simulink library "QuadModelLib"  (R2023a)
settings: Solver=VariableStepAuto  StartTime=0.0  StopTime=10.0  RelTol=1e-3
values from neighbouring files (symbols this model uses):
  ModelParam_envAltitude = -50    [Init.m]
  ModelParam_noisePowerIMU = 0    [Init.m]
  ModelParam_timeSampBaro = 0.01    [Init.m]
  MotorFault1 = MotorFaultTemp    [Init.m]
undefined symbols (not defined in the file or in its folder): BatteryFault, Earth, F, FaultParamAPI, Light, LoadFault, MIL, ModelParam_noiseLowPassFilterCoeAccel, ModelParam_noiseLowPassFilterCoeGyro, Moderate, PropFault, SensorFault, WGS84, WindFault
libraries: aerolibwind2 x4, aerolibtransform2 x1, simulink x1, aerolibasang x1, aerolibatmos2 x1, aerolibnav x1, aerolibgravity2 x1
(part 1 of 2)
settings Model: Creator=dream  LastModifiedBy=RFLYSIM
settings SolverCC: AlgebraicLoopSolver=TrustRegion
settings DataIOCC: ReturnWorkspaceOutputs=off
settings DebuggingCC: UnconnectedInputMsg=warning  UnconnectedOutputMsg=warning  UnconnectedLineMsg=warning  ArithmeticOperatorsInVariantConditions=warning
settings ModelReferenceCC: EnableRefExpFcnMdlSchedulingChecks=on
settings SFSimCC: SimUseLocalCustomCode=off  CustomCodeUndefinedFunction=UseInterfaceOnly
settings RTWCC: RTWUseLocalCustomCode=off  DLArmComputeVersion=19.05

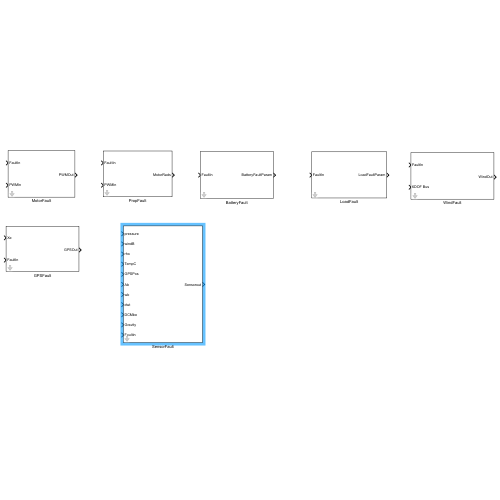
[thumbnail: Simulink's stored preview of the top-level diagram]
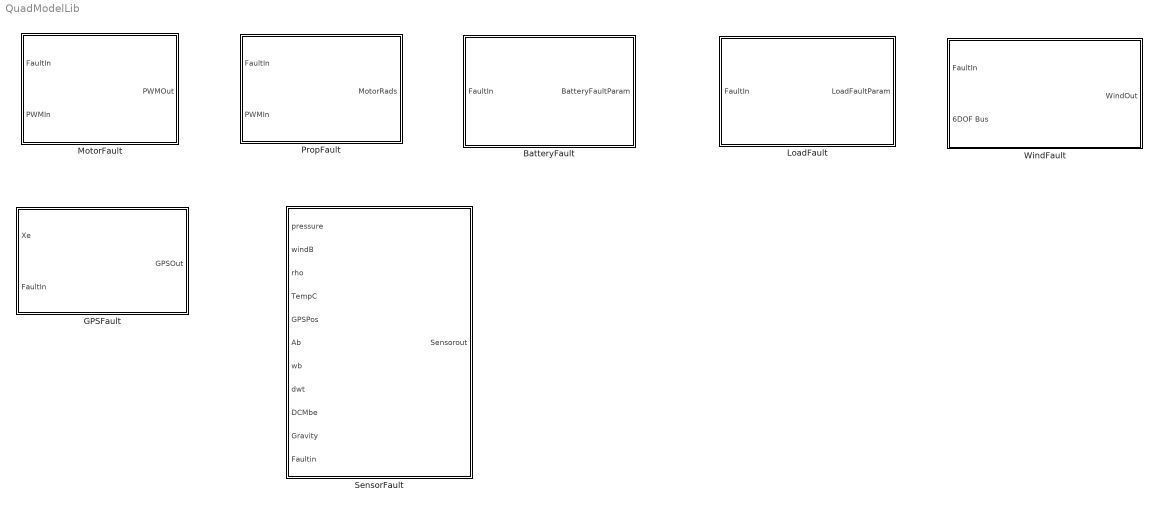
== system QuadModelLib ==
  BatteryFault : Subsystem  mask{FaultParamStruct=BatteryFault}
      mask prompts: FaultParamStruct "Fault Param Struct"
  GPSFault : Subsystem  mask{FaultParamStruct=SensorFault}
      mask prompts: FaultParamStruct "Fault Param Struct"
  LoadFault : Subsystem  mask{FaultParamStruct=LoadFault}
      mask prompts: FaultParamStruct "Fault Param Struct"
  MotorFault : Subsystem  mask{FaultParamStruct=MotorFault1, ComParamVect=FaultParamAPI}
      mask prompts: FaultParamStruct "Fault Param Struct"; ComParamVect "Common Param Vect"
  PropFault : Subsystem  mask{FaultParamStruct=PropFault, ComParamVect=FaultParamAPI}
      mask prompts: FaultParamStruct "Fault Param Struct"; ComParamVect "Common Struct Vect"
  SensorFault : Subsystem  mask{FaultParamStruct=SensorFault, ComParamVect=FaultParamAPI}
      mask prompts: FaultParamStruct "Fault Param Struct"; ComParamVect "Common Param Vect"
  WindFault : Subsystem  mask{FaultParamStruct=WindFault, ComParamVect=FaultParamAPI}
      mask prompts: FaultParamStruct "Fault Param Struct"; ComParamVect "Common Param Vect"

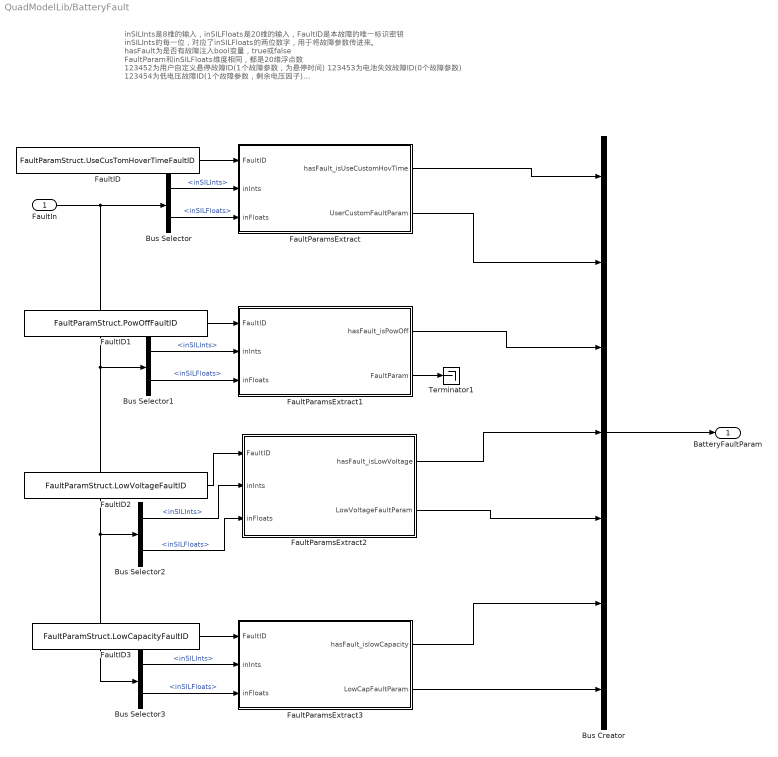
== system QuadModelLib/BatteryFault ==
  note: inSILInts是8维的输入，inSILFloats是20维的输入，FaultID是本故障的唯一标识密钥
      | inSILInts的每一位，对应了inSILFloats的两位数字，用于将故障参数传进来。
      |
      | hasFault为是否有故障注入bool变量，true或false
      | FaultParam和inSILFloats维度相同，都是20维浮点数
      |
      | 123452为用户自定义悬停故障ID(1个故障参数，为悬停时间)
      | 123453为电池失效故障ID(0个故障参数)
      | 123454为低电压故障ID(1个故障参数，剩余电压因子)
      | 123455为低电量故障ID(1个故障参数，剩余电量因子)
      |
      | 注：如果没有新的故障注入进来，FaultParamsExtract会保持上一时刻的值。
  FaultIn : Inport
  Bus Creator : BusCreator  Inputs=7
  Bus Selector{,1..3} (4 alike) : BusSelector  OutputSignals=inSILInts,inSILFloats
  FaultID : Constant  Value=FaultParamStruct.UseCusTomHoverTimeFaultID  OutDataTypeStr=int32
  FaultID1 : Constant  Value=FaultParamStruct.PowOffFaultID  OutDataTypeStr=int32
  FaultID2 : Constant  Value=FaultParamStruct.LowVoltageFaultID  OutDataTypeStr=int32
  FaultID3 : Constant  Value=FaultParamStruct.LowCapacityFaultID  OutDataTypeStr=int32
  FaultParamsExtract : MATLAB Function  TreatAsAtomicUnit=on
  FaultParamsExtract1 : MATLAB Function  TreatAsAtomicUnit=on
  FaultParamsExtract2 : MATLAB Function  TreatAsAtomicUnit=on
  FaultParamsExtract3 : MATLAB Function  TreatAsAtomicUnit=on
  Terminator1 : Terminator
  BatteryFaultParam : Outport
  wires:
  Bus Selector3/2 -> FaultParamsExtract3/3(inFloats)  "<inSILFloats>"
  Bus Selector3/1 -> FaultParamsExtract3/2(inInts)  "<inSILInts>"
  FaultIn/1 -> Bus Selector/1, Bus Selector3/1, Bus Selector2/1, Bus Selector1/1
  Bus Selector1/1 -> FaultParamsExtract1/2(inInts)  "<inSILInts>"
  Bus Selector2/1 -> FaultParamsExtract2/2(inInts)  "<inSILInts>"
  FaultParamsExtract2/2(LowVoltageFaultParam) -> Bus Creator/5
  Bus Selector/1 -> FaultParamsExtract/2(inInts)  "<inSILInts>"
  FaultID2/1 -> FaultParamsExtract2/1(FaultID)
  FaultParamsExtract3/2(LowCapFaultParam) -> Bus Creator/7
  Bus Selector1/2 -> FaultParamsExtract1/3(inFloats)  "<inSILFloats>"
  FaultParamsExtract/2(UserCustomFaultParam) -> Bus Creator/2
  FaultID1/1 -> FaultParamsExtract1/1(FaultID)
  FaultID3/1 -> FaultParamsExtract3/1(FaultID)
  Bus Selector2/2 -> FaultParamsExtract2/3(inFloats)  "<inSILFloats>"
  FaultParamsExtract1/2(FaultParam) -> Terminator1/1
  Bus Selector/2 -> FaultParamsExtract/3(inFloats)  "<inSILFloats>"
  FaultID/1 -> FaultParamsExtract/1(FaultID)
  FaultParamsExtract1/1(hasFault_isPowOff) -> Bus Creator/3
  FaultParamsExtract/1(hasFault_isUseCustomHovTime) -> Bus Creator/1
  FaultParamsExtract2/1(hasFault_isLowVoltage) -> Bus Creator/4
  FaultParamsExtract3/1(hasFault_islowCapacity) -> Bus Creator/6
  Bus Creator/1 -> BatteryFaultParam/1

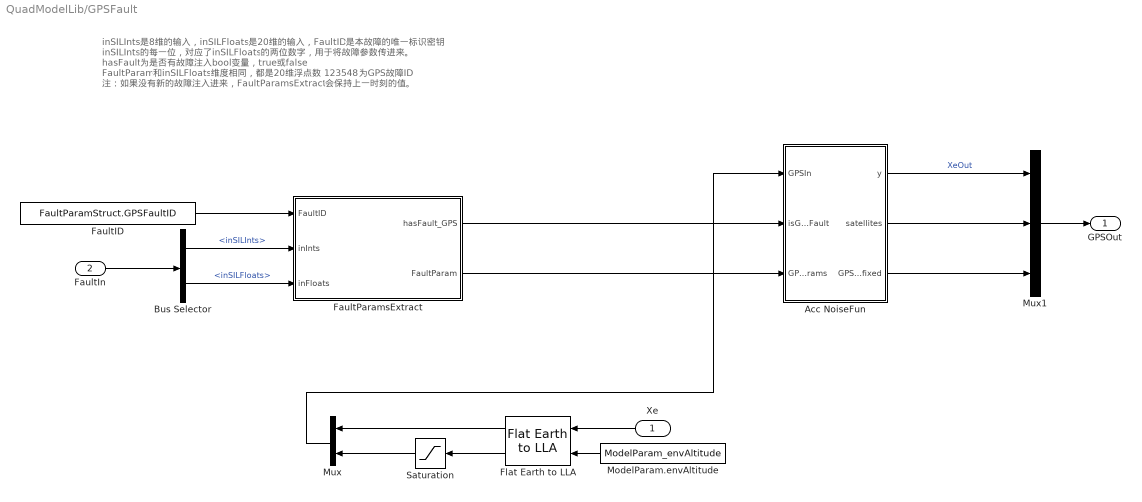
== system QuadModelLib/GPSFault ==
  note: inSILInts是8维的输入，inSILFloats是20维的输入，FaultID是本故障的唯一标识密钥
      | inSILInts的每一位，对应了inSILFloats的两位数字，用于将故障参数传进来。
      |
      | hasFault为是否有故障注入bool变量，true或false
      | FaultParam和inSILFloats维度相同，都是20维浮点数
      |
      | 123548为GPS故障ID
      |
      | 注：如果没有新的故障注入进来，FaultParamsExtract会保持上一时刻的值。
  Xe : Inport
  FaultIn : Inport  Port=2
  Acc NoiseFun : MATLAB Function  TreatAsAtomicUnit=on
  Bus Selector : BusSelector  OutputSignals=inSILInts,inSILFloats
  FaultID : Constant  Value=FaultParamStruct.GPSFaultID  OutDataTypeStr=int32
  FaultParamsExtract : MATLAB Function  TreatAsAtomicUnit=on
  Flat Earth to LLA : aerolibtransform2/Flat Earth to LLA  units=Metric (MKS)  ptype=Earth (WGS84)  F=1/298.257223563  R=6378137  refPosPort=off  LL0=ModelParam_GPSLatLong  psi=0
  ModelParam.envAltitude : Constant  Value=ModelParam_envAltitude
  Mux : Mux  Inputs=2
  Mux1 : Mux  Inputs=3
  Saturation : Saturate  UpperLimit=100000  LowerLimit=0
  GPSOut : Outport
  wires:
  FaultParamsExtract/1(hasFault_GPS) -> Acc NoiseFun/2(isGPSFault)
  Bus Selector/2 -> FaultParamsExtract/3(inFloats)  "<inSILFloats>"
  FaultID/1 -> FaultParamsExtract/1(FaultID)
  FaultIn/1 -> Bus Selector/1
  FaultParamsExtract/2(FaultParam) -> Acc NoiseFun/3(GPSFaultParams)
  Flat Earth to LLA/2 -> Saturation/1
  ModelParam.envAltitude/1 -> Flat Earth to LLA/2
  Flat Earth to LLA/1 -> Mux/1
  Saturation/1 -> Mux/2
  Bus Selector/1 -> FaultParamsExtract/2(inInts)  "<inSILInts>"
  Acc NoiseFun/2(satellites) -> Mux1/2
  Acc NoiseFun/3(GPS3Dfixed) -> Mux1/3
  Mux1/1 -> GPSOut/1
  Xe/1 -> Flat Earth to LLA/1
  Mux/1 -> Acc NoiseFun/1(GPSIn)
  Acc NoiseFun/1(y) -> Mux1/1  "XeOut"

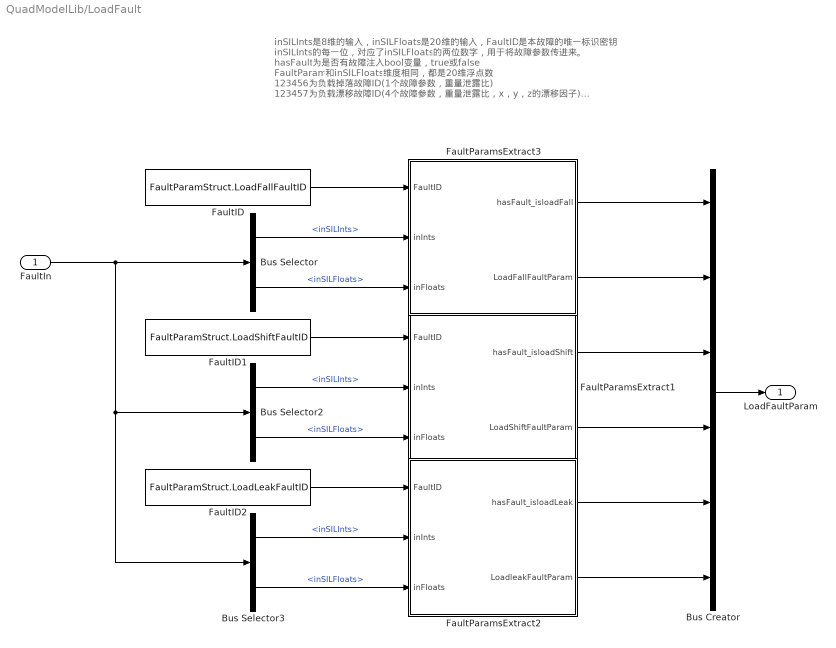
== system QuadModelLib/LoadFault ==
  note: inSILInts是8维的输入，inSILFloats是20维的输入，FaultID是本故障的唯一标识密钥
      | inSILInts的每一位，对应了inSILFloats的两位数字，用于将故障参数传进来。
      |
      | hasFault为是否有故障注入bool变量，true或false
      | FaultParam和inSILFloats维度相同，都是20维浮点数
      |
      | 123456为负载掉落故障ID(1个故障参数，重量泄露比)
      | 123457为负载漂移故障ID(4个故障参数，重量泄露比，x，y，z的漂移因子)
      | 123458为负载泄露故障ID(2个故障参数，1个重量泄露比，1个泄露因子)
      | 注：如果没有新的故障注入进来，FaultParamsExtract会保持上一时刻的值。
  FaultIn : Inport
  Bus Creator : BusCreator  Inputs=6
  Bus Selector : BusSelector  OutputSignals=inSILInts,inSILFloats
  Bus Selector2 : BusSelector  OutputSignals=inSILInts,inSILFloats
  Bus Selector3 : BusSelector  OutputSignals=inSILInts,inSILFloats
  FaultID : Constant  Value=FaultParamStruct.LoadFallFaultID  OutDataTypeStr=int32
  FaultID1 : Constant  Value=FaultParamStruct.LoadShiftFaultID  OutDataTypeStr=int32
  FaultID2 : Constant  Value=FaultParamStruct.LoadLeakFaultID  OutDataTypeStr=int32
  FaultParamsExtract1 : MATLAB Function  TreatAsAtomicUnit=on
  FaultParamsExtract2 : MATLAB Function  TreatAsAtomicUnit=on
  FaultParamsExtract3 : MATLAB Function  TreatAsAtomicUnit=on
  LoadFaultParam : Outport
  wires:
  FaultIn/1 -> Bus Selector3/1, Bus Selector2/1, Bus Selector/1
  Bus Selector3/2 -> FaultParamsExtract2/3(inFloats)  "<inSILFloats>"
  Bus Selector/1 -> FaultParamsExtract3/2(inInts)  "<inSILInts>"
  Bus Selector2/2 -> FaultParamsExtract1/3(inFloats)  "<inSILFloats>"
  Bus Selector3/1 -> FaultParamsExtract2/2(inInts)  "<inSILInts>"
  Bus Selector2/1 -> FaultParamsExtract1/2(inInts)  "<inSILInts>"
  Bus Selector/2 -> FaultParamsExtract3/3(inFloats)  "<inSILFloats>"
  FaultID/1 -> FaultParamsExtract3/1(FaultID)
  FaultID2/1 -> FaultParamsExtract2/1(FaultID)
  FaultID1/1 -> FaultParamsExtract1/1(FaultID)
  FaultParamsExtract3/1(hasFault_isloadFall) -> Bus Creator/1
  FaultParamsExtract3/2(LoadFallFaultParam) -> Bus Creator/2
  FaultParamsExtract1/1(hasFault_isloadShift) -> Bus Creator/3
  FaultParamsExtract1/2(LoadShiftFaultParam) -> Bus Creator/4
  FaultParamsExtract2/1(hasFault_isloadLeak) -> Bus Creator/5
  FaultParamsExtract2/2(LoadleakFaultParam) -> Bus Creator/6
  Bus Creator/1 -> LoadFaultParam/1

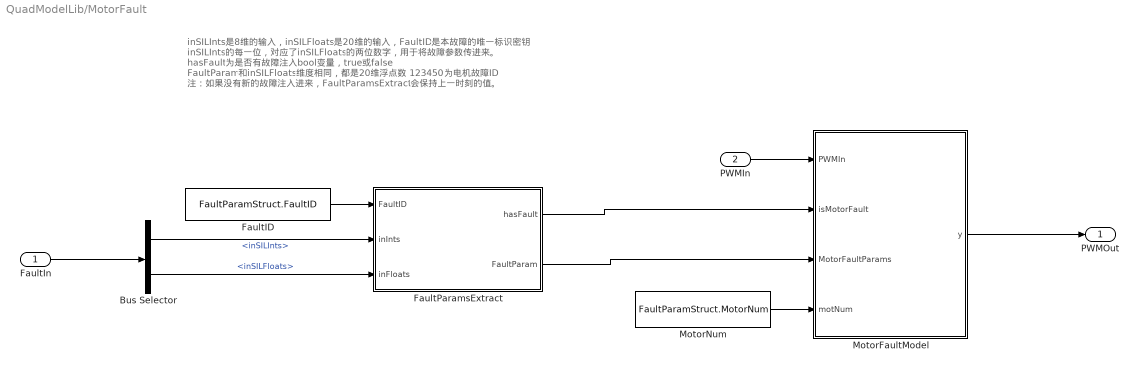
== system QuadModelLib/MotorFault ==
  note: inSILInts是8维的输入，inSILFloats是20维的输入，FaultID是本故障的唯一标识密钥
      | inSILInts的每一位，对应了inSILFloats的两位数字，用于将故障参数传进来。
      |
      | hasFault为是否有故障注入bool变量，true或false
      | FaultParam和inSILFloats维度相同，都是20维浮点数
      |
      | 123450为电机故障ID
      |
      | 注：如果没有新的故障注入进来，FaultParamsExtract会保持上一时刻的值。
  FaultIn : Inport
  PWMIn : Inport  Port=2
  Bus Selector : BusSelector  OutputSignals=inSILInts,inSILFloats
  FaultID : Constant  Value=FaultParamStruct.FaultID  OutDataTypeStr=int32
  FaultParamsExtract : MATLAB Function  TreatAsAtomicUnit=on
  MotorFaultModel : MATLAB Function  TreatAsAtomicUnit=on
  MotorNum : Constant  Value=FaultParamStruct.MotorNum  OutDataTypeStr=int32
  PWMOut : Outport
  wires:
  FaultIn/1 -> Bus Selector/1
  FaultID/1 -> FaultParamsExtract/1(FaultID)
  MotorFaultModel/1(y) -> PWMOut/1
  Bus Selector/2 -> FaultParamsExtract/3(inFloats)  "<inSILFloats>"
  MotorNum/1 -> MotorFaultModel/4(motNum)
  Bus Selector/1 -> FaultParamsExtract/2(inInts)  "<inSILInts>"
  PWMIn/1 -> MotorFaultModel/1(PWMIn)
  FaultParamsExtract/1(hasFault) -> MotorFaultModel/2(isMotorFault)
  FaultParamsExtract/2(FaultParam) -> MotorFaultModel/3(MotorFaultParams)

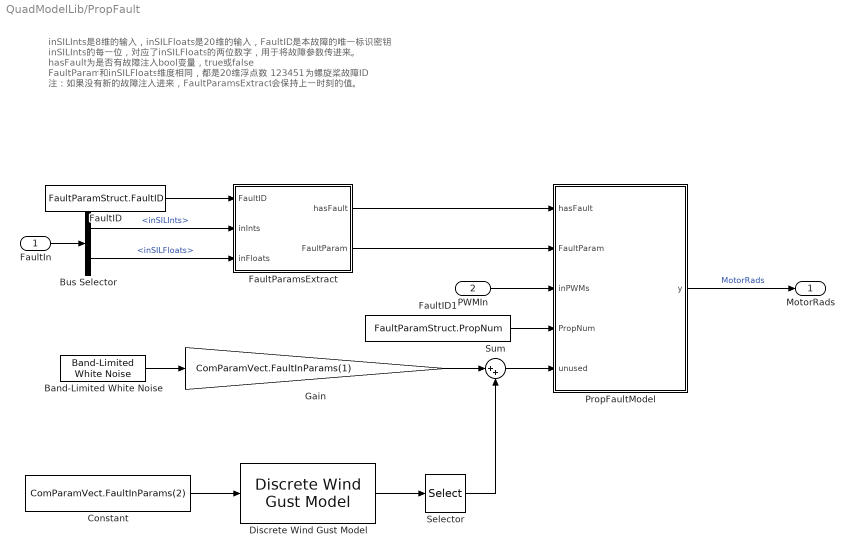
== system QuadModelLib/PropFault ==
  note: inSILInts是8维的输入，inSILFloats是20维的输入，FaultID是本故障的唯一标识密钥
      | inSILInts的每一位，对应了inSILFloats的两位数字，用于将故障参数传进来。
      |
      | hasFault为是否有故障注入bool变量，true或false
      | FaultParam和inSILFloats维度相同，都是20维浮点数
      |
      | 123451为螺旋桨故障ID
      | 注：如果没有新的故障注入进来，FaultParamsExtract会保持上一时刻的值。
  FaultIn : Inport
  PWMIn : Inport  Port=2
  Band-Limited White Noise : simulink/Sources/Band-Limited White Noise  Cov=[1]  Ts=0.1  seed=[23341]
  Bus Selector : BusSelector  OutputSignals=inSILInts,inSILFloats
  Constant : Constant  Value=ComParamVect.FaultInParams(2)
  Discrete Wind Gust Model : aerolibwind2/Discrete Wind Gust Model  units=Metric (MKS)  Gx=on  Gy=on  Gz=on  t_0=ComParamVect.FaultInParams(3)  d_m=[120 120 80]  v_m=[3.5 3.5 3.0]
  FaultID : Constant  Value=FaultParamStruct.FaultID  OutDataTypeStr=int32
  FaultID1 : Constant  Value=FaultParamStruct.PropNum  OutDataTypeStr=int32
  FaultParamsExtract : MATLAB Function  TreatAsAtomicUnit=on
  Gain : Gain  Gain=ComParamVect.FaultInParams(1)
  PropFaultModel : MATLAB Function  TreatAsAtomicUnit=on
  Selector : Selector  InputPortWidth=3  IndexOptions=Index vector (dialog)  Indices=[1]  OutputSizes=1
  Sum : Sum  Inputs=|++
  MotorRads : Outport  VectorParamsAs1DForOutWhenUnconnected=off
  wires:
  FaultParamsExtract/1(hasFault) -> PropFaultModel/1(hasFault)
  Bus Selector/2 -> FaultParamsExtract/3(inFloats)  "<inSILFloats>"
  FaultID/1 -> FaultParamsExtract/1(FaultID)
  Bus Selector/1 -> FaultParamsExtract/2(inInts)  "<inSILInts>"
  FaultParamsExtract/2(FaultParam) -> PropFaultModel/2(FaultParam)
  PWMIn/1 -> PropFaultModel/3(inPWMs)
  PropFaultModel/1(y) -> MotorRads/1  "MotorRads"
  FaultIn/1 -> Bus Selector/1
  FaultID1/1 -> PropFaultModel/4(PropNum)
  Sum/1 -> PropFaultModel/5(unused)
  Gain/1 -> Sum/1
  Discrete Wind Gust Model/1 -> Selector/1
  Band-Limited White Noise/1 -> Gain/1
  Selector/1 -> Sum/2
  Constant/1 -> Discrete Wind Gust Model/1

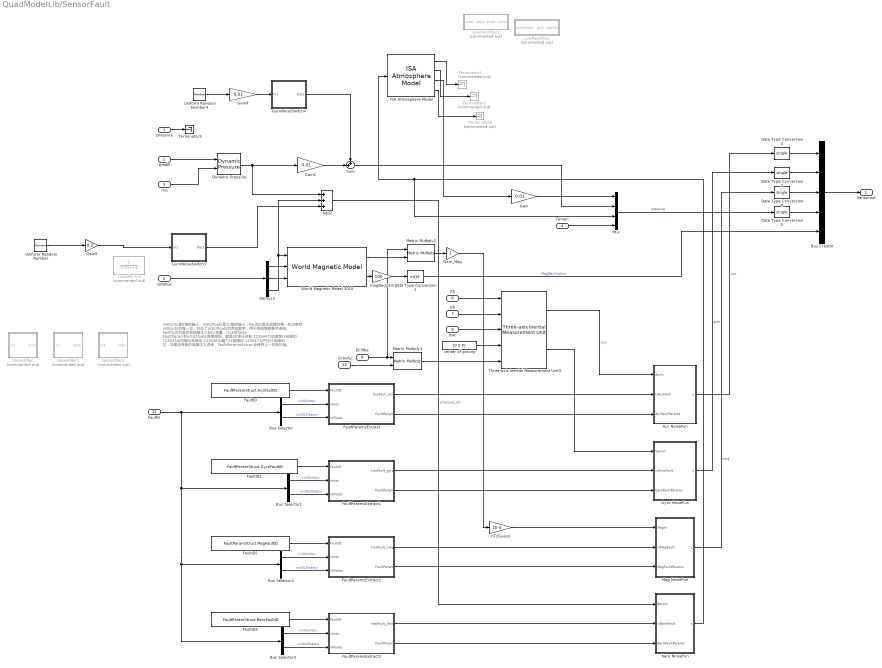
== system QuadModelLib/SensorFault ==
  note: inSILInts是8维的输入，inSILFloats是20维的输入，FaultID是本故障的唯一标识密钥
      | inSILInts的每一位，对应了inSILFloats的两位数字，用于将故障参数传进来。
      |
      | hasFault为是否有故障注入bool变量，true或false
      | FaultParam和inSILFloats维度相同，都是20维浮点数
      |
      | 123544为加速度计故障ID
      | 123545为陀螺仪故障ID
      | 123546为磁力计故障ID
      | 123547为气压计故障ID
      | 注：如果没有新的故障注入进来，FaultParamsExtract会保持上一时刻的值。
  pressure : Inport
  windB : Inport  Port=2
  rho : Inport  Port=3
  TempC : Inport  Port=4
  GPSPos : Inport  Port=5
  Ab : Inport  Port=6
  wb : Inport  Port=7
  dwt : Inport  Port=8
  DCMbe : Inport  Port=9
  Gravity : Inport  Port=10
  Faultin : Inport  Port=11
  Acc NoiseFun : MATLAB Function  TreatAsAtomicUnit=on
  Add2 : Sum  Inputs=+++
  Bus Creator : BusCreator  Inputs=5
  Bus Selector{,1..3} (4 alike) : BusSelector  OutputSignals=inSILInts,inSILFloats
  Data Type Conversion1 : DataTypeConversion  OutDataTypeStr=int16  SaturateOnIntegerOverflow=off  RndMeth=Floor
  Data Type Conversion{2..5} (4 alike) : DataTypeConversion  OutDataTypeStr=single  SaturateOnIntegerOverflow=off  RndMeth=Floor
  Demux2 : Demux  Outputs=3
  Dynamic Pressure : aerolibasang/Dynamic Pressure
  FaultID : Constant  Value=FaultParamStruct.AccFaultID  OutDataTypeStr=int32
  FaultID1 : Constant  Value=FaultParamStruct.GyroFaultID  OutDataTypeStr=int32
  FaultID2 : Constant  Value=FaultParamStruct.MagFaultID  OutDataTypeStr=int32
  FaultID3 : Constant  Value=FaultParamStruct.BaroFaultID  OutDataTypeStr=int32
  FaultParamsExtract : MATLAB Function  TreatAsAtomicUnit=on
  FaultParamsExtract1 : MATLAB Function  TreatAsAtomicUnit=on
  FaultParamsExtract2 : MATLAB Function  TreatAsAtomicUnit=on
  FaultParamsExtract3 : MATLAB Function  TreatAsAtomicUnit=on
  Gain : Gain  Gain=0.01
  Gain1 : Gain  Gain=0.01
  Gain5 : Gain  Gain=0.2
  Gain9 : Gain  Gain=0.01
  Gain_Mag : Gain
  Gyro NoiseFun : MATLAB Function  TreatAsAtomicUnit=on
  GyroNoiseSwitch3 : Subsystem
  GyroNoiseSwitch4 : Subsystem
  ISA Atmosphere Model : aerolibatmos2/ISA Atmosphere Model  custom=off  g=9.80665  gamma=1.4  R=287.0531  L=0.0065  h_trop=11000  h_strat=20000  rho0=1.225  P0=101325  T0=288.15  h0=0
  LowPassFilter : Subsystem  Commented=on
  LowPassFilter2 : Subsystem  Commented=on
  Mag NoiseFun : MATLAB Function  TreatAsAtomicUnit=on
  Matrix Multiply1 : Product  Multiplication=Matrix(*)
  Matrix Multiply2 : Product  Multiplication=Matrix(*)
  Mux : Mux
  NoiseFilter : Subsystem  Commented=on
  NoiseFilter1 : Subsystem  Commented=on
  NoiseFilter2 : Subsystem  Commented=on
  Sum : Sum  Inputs=++|
  Terminator1 : Terminator  Commented=on
  Terminator2 : Terminator  Commented=on
  Terminator3 : Terminator
  Terminator4 : Terminator  Commented=on
  Three-axis Inertial Measurement Unit3 : aerolibnav/Three-axis Inertial Measurement Unit  units=Metric (MKS)  imu=[0 0 0]  i_Ts=0  dtype_a=on  w_a=190  z_a=ComParamVect.FaultInParams(10)  a_sf_cc=[1 0 0; 0 1 0; 0 0 1]  a_bias=[ComParamVect.FaultInParams(11) ComParamVect.FaultInParams(12) ComParamVect.FaultInParams(13)]  a_sat="[-160  -160  -160 160 160 160]"  dtype_g=on  w_g=190  z_g=ComParamVect.FaultInParams(14)  g_sf_cc=[1 0 0; 0 1 0; 0 0 1]  g_bias=[ComParamVect.FaultInParams(15) ComParamVect.FaultInParams(16) ComParamVect.FaultInParams(17)]  g_sens=[0 0 0]  g_sat="[-4.36  -4.36  -4.36 4.36 4.36 4.36]"  i_rand=off  i_seeds=[23093 23094 23095 23096 23097 23098]  i_pow=ModelParam_noisePowerIMU*[0.0000005 0.0000005 0.0000005 0.000000002 0.000000002 0.000000002]
  Transfer Fcn : TransferFcn  Commented=on  Denominator=[0.05 1]
  Uniform Random Number : UniformRandomNumber  Minimum=-2  Maximum=2  Seed=15634  SampleTime=ModelParam_timeSampBaro
  Uniform Random Number4 : UniformRandomNumber  Seed=25634  SampleTime=0.01
  World Magnetic Model 2015 : aerolibgravity2/World Magnetic Model  model=WMM2015 V2 (2015-2020)  customFile='WMM2020.COF'  units=Metric (MKS)  time_in=off  month=November  day=3  year=2017  action=Error  h_out=off  dec_out=on  inc_out=off  ti_out=off
  baro NoiseFun : MATLAB Function  TreatAsAtomicUnit=on
  center of gravity : Constant  Value=[0 0 0]
  magDecGain : Gain  Gain=100
  nT2Gauss : Gain  Gain=1E-5
  Sensorout : Outport
  wires:
  FaultParamsExtract3/2(FaultParam) -> baro NoiseFun/3(BaroFaultParams)
  Gain9/1 -> GyroNoiseSwitch4/1(In1)
  Matrix Multiply1/1 -> Three-axis Inertial Measurement Unit3/5
  FaultParamsExtract1/1(hasFault_gyro) -> Gyro NoiseFun/2(isGyroFault)
  FaultParamsExtract1/2(FaultParam) -> Gyro NoiseFun/3(GyroFaultParams)
  FaultParamsExtract/1(hasFault_acc) -> Acc NoiseFun/2(isAccFault)
  Bus Selector3/1 -> FaultParamsExtract3/2(inInts)  "<inSILInts>"
  Mux/1 -> Data Type Conversion5/1  "pressure"
  FaultID/1 -> FaultParamsExtract/1(FaultID)
  Sum/1 -> Mux/2
  wb/1 -> Three-axis Inertial Measurement Unit3/2
  TempC/1 -> Mux/4
  nT2Gauss/1 -> Mag NoiseFun/1(MagIn)
  center of gravity/1 -> Three-axis Inertial Measurement Unit3/4
  Gravity/1 -> Matrix Multiply1/2
  Bus Selector1/2 -> FaultParamsExtract1/3(inFloats)  "<inSILFloats>"
  Ab/1 -> Three-axis Inertial Measurement Unit3/1
  FaultID2/1 -> FaultParamsExtract2/1(FaultID)
  World Magnetic Model 2015/1 -> Matrix Multiply2/2
  Bus Selector3/2 -> FaultParamsExtract3/3(inFloats)  "<inSILFloats>"
  magDecGain/1 -> Data Type Conversion1/1
  DCMbe/1 -> Matrix Multiply2/1, Matrix Multiply1/1
  Three-axis Inertial Measurement Unit3/2 -> Gyro NoiseFun/1(GyroIn)
  Gain_Mag/1 -> nT2Gauss/1
  Bus Selector1/1 -> FaultParamsExtract1/2(inInts)  "<inSILInts>"
  ISA Atmosphere Model/3 -> Gain/1
  Gain1/1 -> Sum/2
  Bus Selector/2 -> FaultParamsExtract/3(inFloats)  "<inSILFloats>"
  FaultParamsExtract3/1(hasFault_baro) -> baro NoiseFun/2(isBaroFault)
  FaultID1/1 -> FaultParamsExtract1/1(FaultID)
  ISA Atmosphere Model/1 -> Terminator1/1
  Gain/1 -> Mux/1
  pressure/1 -> Terminator3/1
  Demux2/1 -> World Magnetic Model 2015/2
  Bus Selector2/1 -> FaultParamsExtract2/2(inInts)  "<inSILInts>"
  Uniform Random Number4/1 -> Gain9/1
  GyroNoiseSwitch4/1(Out1) -> Sum/1
  ISA Atmosphere Model/2 -> Terminator2/1
  windB/1 -> Dynamic Pressure/1
  FaultID3/1 -> FaultParamsExtract3/1(FaultID)
  GPSPos/1 -> Demux2/1
  Uniform Random Number/1 -> Gain5/1
  Bus Selector/1 -> FaultParamsExtract/2(inInts)  "<inSILInts>"
  dwt/1 -> Three-axis Inertial Measurement Unit3/3
  FaultParamsExtract2/2(FaultParam) -> Mag NoiseFun/3(MagFaultParams)
  World Magnetic Model 2015/2 -> magDecGain/1
  GyroNoiseSwitch3/1(Out1) -> Add2/3
  Faultin/1 -> Bus Selector3/1, Bus Selector2/1, Bus Selector1/1, Bus Selector/1
  Demux2/3 -> World Magnetic Model 2015/1, Add2/2
  Bus Selector2/2 -> FaultParamsExtract2/3(inFloats)  "<inSILFloats>"
  Gyro NoiseFun/1(y) -> Data Type Conversion3/1  "gyro"
  Acc NoiseFun/1(y) -> Data Type Conversion2/1  "acc"
  Matrix Multiply2/1 -> Gain_Mag/1
  Mag NoiseFun/1(y) -> Data Type Conversion4/1  "mag"
  Dynamic Pressure/1 -> Add2/1, Gain1/1
  ISA Atmosphere Model/4 -> Terminator4/1
  FaultParamsExtract2/1(hasFault_mag) -> Mag NoiseFun/2(isMagFault)
  Gain5/1 -> GyroNoiseSwitch3/1(In1)
  Demux2/2 -> World Magnetic Model 2015/3
  FaultParamsExtract/2(FaultParam) -> Acc NoiseFun/3(AccFaultParams)
  rho/1 -> Dynamic Pressure/2
  Data Type Conversion1/1 -> Bus Creator/5  "MagDeclination"
  Bus Creator/1 -> Sensorout/1
  Data Type Conversion2/1 -> Bus Creator/1
  Data Type Conversion3/1 -> Bus Creator/2
  Data Type Conversion4/1 -> Bus Creator/3
  Data Type Conversion5/1 -> Bus Creator/4
  Add2/1 -> baro NoiseFun/1(BaroIn)  "pressure_alt"
  baro NoiseFun/1(y) -> Mux/3, ISA Atmosphere Model/1
  Three-axis Inertial Measurement Unit3/1 -> Acc NoiseFun/1(AccIn)  "acc"

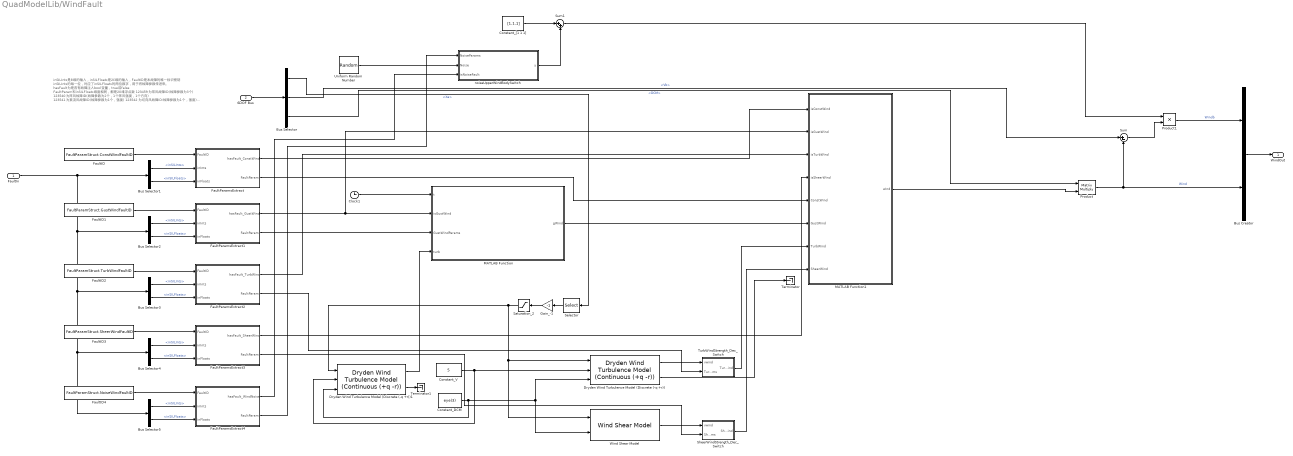
== system QuadModelLib/WindFault ==
  note: inSILInts是8维的输入，inSILFloats是20维的输入，FaultID是本故障的唯一标识密钥
      | inSILInts的每一位，对应了inSILFloats的两位数字，用于将故障参数传进来。
      |
      | hasFault为是否有故障注入bool变量，true或false
      | FaultParam和inSILFloats维度相同，都是20维浮点数
      |
      | 123459为常风故障ID(故障参数为3个)
      | 123540为阵风故障ID(故障参数为2个，1个阵风强度，1个方向)
      | 123541为紊流风故障ID(故障参数为1个，强度)
      | 123542为切向风故障ID(故障参数为1个，强度)
      | 123543为噪声风故障ID(参数为2个，1格式风振幅扰动因子范围0到1,1个风增益水平）)
      | 注：如果没有新的故障注入进来，FaultParamsExtract会保持上一时刻的值。
  FaultIn : Inport
  6DOF Bus : Inport  Port=2
  Bus Creator : BusCreator  Inputs=2
  Bus Selector : BusSelector  OutputSignals=Xe,Vb,DCM
  Bus Selector{1..5} (5 alike) : BusSelector  OutputSignals=inSILInts,inSILFloats
  Clock1 : Clock
  Constant_DCM : Constant  Value=eye(3)
  Constant_V : Constant  Value=5
  Constant_[1 1 1] : Constant  Value=[1,1,1]  VectorParams1D=off
  Dryden Wind Turbulence Model (Discrete (-q +r)) : aerolibwind2/Dryden Wind Turbulence Model  (Continuous (+q -r))  units=Metric (MKS)  spec=MIL-F-8785C  model=Discrete Dryden (-q +r)  W20=ComParamVect.FaultInParams(4)  Wdeg=ComParamVect.FaultInParams(5)  TurbProb=10^-3 - Moderate  L_high=533.4  Wingspan=1  ts=ModelParam_timeSampTurbWind  Seed=[23341 23342 23343 23344]  T_on=on
  Dryden Wind Turbulence Model (Discrete (-q +r))1 : aerolibwind2/Dryden Wind Turbulence Model  (Continuous (+q -r))  units=Metric (MKS)  spec=MIL-F-8785C  model=Discrete Dryden (-q +r)  W20=ComParamVect.FaultInParams(8)  Wdeg=ComParamVect.FaultInParams(9)  TurbProb=10^-2 - Light  L_high=533.4  Wingspan=1  ts=ModelParam_timeSampTurbWind  Seed=[23301 23542 82443 33344]  T_on=on
  FaultID : Constant  Value=FaultParamStruct.ConstWindFaultID  OutDataTypeStr=int32
  FaultID1 : Constant  Value=FaultParamStruct.GustWindFaultID  OutDataTypeStr=int32
  FaultID2 : Constant  Value=FaultParamStruct.TurbWindFaultID  OutDataTypeStr=int32
  FaultID3 : Constant  Value=FaultParamStruct.SheerWindFaultID  OutDataTypeStr=int32
  FaultID4 : Constant  Value=FaultParamStruct.NoiseWindFaultID  OutDataTypeStr=int32
  FaultParamsExtract : MATLAB Function  TreatAsAtomicUnit=on
  FaultParamsExtract1 : MATLAB Function  TreatAsAtomicUnit=on
  FaultParamsExtract2 : MATLAB Function  TreatAsAtomicUnit=on
  FaultParamsExtract3 : MATLAB Function  TreatAsAtomicUnit=on
  FaultParamsExtract4 : MATLAB Function  TreatAsAtomicUnit=on
  Gain_-1 : Gain  Gain=-1
  MATLAB Function : MATLAB Function  TreatAsAtomicUnit=on
  MATLAB Function1 : MATLAB Function  TreatAsAtomicUnit=on
  Product : Product  Multiplication=Matrix(*)
  Product1 : Product
  Saturation_2 : Saturate  UpperLimit=10000  LowerLimit=0
  Selector : Selector  InputPortWidth=3  IndexOptions=Index vector (dialog)  Indices=[3]  OutputSizes=1
  SheerWindStrength_Dec_Switch : MATLAB Function  TreatAsAtomicUnit=on
  Sum : Sum  Inputs=|+-
  Sum1 : Sum  Inputs=|++
  Terminator : Terminator
  Terminator1 : Terminator
  TurbWindStrength_Dec_Switch : MATLAB Function  TreatAsAtomicUnit=on
  Uniform Random Number : UniformRandomNumber  Minimum=[-1,-1,-0.5]  Maximum=[1,1,0.5]  Seed=[564565,6846798,46545]  SampleTime=0.003
  Wind Shear Model : aerolibwind2/Wind Shear Model  units=Metric (MKS)  phase=Category C - Terminal Flight Phase  W_20=ComParamVect.FaultInParams(6)  Wdeg=ComParamVect.FaultInParams(7)
  noiseUpperWindBodySwitch : MATLAB Function  TreatAsAtomicUnit=on
  WindOut : Outport
  wires:
  Product/1 -> Bus Creator/2, Sum/2  "Wind"
  Constant_DCM/1 -> Dryden Wind Turbulence Model (Discrete (-q +r))/3, Wind Shear Model/2, Dryden Wind Turbulence Model (Discrete (-q +r))1/3
  Clock1/1 -> MATLAB Function/1(t)
  FaultParamsExtract2/2(FaultParam) -> TurbWindStrength_Dec_Switch/2(TurbWindParams)
  FaultID1/1 -> FaultParamsExtract1/1(FaultID)
  FaultIn/1 -> Bus Selector5/1, Bus Selector4/1, Bus Selector3/1, Bus Selector2/1, Bus Selector1/1
  Bus Selector2/2 -> FaultParamsExtract1/3(inFloats)  "<inSILFloats>"
  Bus Selector1/2 -> FaultParamsExtract/3(inFloats)  "<inSILFloats>"
  MATLAB Function/1(gWind) -> MATLAB Function1/6(GustWind)
  FaultID2/1 -> FaultParamsExtract2/1(FaultID)
  Sum1/1 -> Product1/1
  FaultID4/1 -> FaultParamsExtract4/1(FaultID)
  Uniform Random Number/1 -> noiseUpperWindBodySwitch/2(Noise)
  Bus Selector1/1 -> FaultParamsExtract/2(inInts)  "<inSILInts>"
  FaultParamsExtract/2(FaultParam) -> MATLAB Function1/5(ConstWind)
  FaultParamsExtract4/1(hasFault_WindNoise) -> noiseUpperWindBodySwitch/3(isNoiseFault)
  Dryden Wind Turbulence Model (Discrete (-q +r))1/1 -> MATLAB Function/4(turb)
  Bus Selector5/2 -> FaultParamsExtract4/3(inFloats)  "<inSILFloats>"
  noiseUpperWindBodySwitch/1(y) -> Sum1/2
  FaultParamsExtract1/1(hasFault_GustWind) -> MATLAB Function/2(isGustWind), MATLAB Function1/2(isGustWind)
  Dryden Wind Turbulence Model (Discrete (-q +r))/2 -> Terminator/1
  Bus Selector3/2 -> FaultParamsExtract2/3(inFloats)  "<inSILFloats>"
  FaultParamsExtract3/1(hasFault_SheerWind) -> MATLAB Function1/4(isSheerWind)
  SheerWindStrength_Dec_Switch/1(SheerWind) -> MATLAB Function1/8(SheerWind)
  Bus Selector4/2 -> FaultParamsExtract3/3(inFloats)  "<inSILFloats>"
  Dryden Wind Turbulence Model (Discrete (-q +r))/1 -> TurbWindStrength_Dec_Switch/1(vwind)
  Bus Selector3/1 -> FaultParamsExtract2/2(inInts)  "<inSILInts>"
  Sum/1 -> Product1/2
  FaultParamsExtract3/2(FaultParam) -> SheerWindStrength_Dec_Switch/2(SheerWindParams)
  FaultID/1 -> FaultParamsExtract/1(FaultID)
  Wind Shear Model/1 -> SheerWindStrength_Dec_Switch/1(vwind)
  FaultParamsExtract4/2(FaultParam) -> noiseUpperWindBodySwitch/1(NoiseParams)
  Dryden Wind Turbulence Model (Discrete (-q +r))1/2 -> Terminator1/1
  Constant_[1 1 1]/1 -> Sum1/1
  Constant_V/1 -> Dryden Wind Turbulence Model (Discrete (-q +r))1/2, Dryden Wind Turbulence Model (Discrete (-q +r))/2
  MATLAB Function1/1(wind) -> Product/2
  FaultParamsExtract2/1(hasFault_TurbWind) -> MATLAB Function1/3(isTurbWind)
  FaultParamsExtract1/2(FaultParam) -> MATLAB Function/3(GustWindParams)
  TurbWindStrength_Dec_Switch/1(TurbWind) -> MATLAB Function1/7(TurbWind)
  Bus Selector4/1 -> FaultParamsExtract3/2(inInts)  "<inSILInts>"
  FaultID3/1 -> FaultParamsExtract3/1(FaultID)
  FaultParamsExtract/1(hasFault_ConstWind) -> MATLAB Function1/1(isConstWind)
  Bus Selector2/1 -> FaultParamsExtract1/2(inInts)  "<inSILInts>"
  Bus Selector5/1 -> FaultParamsExtract4/2(inInts)  "<inSILInts>"
  Bus Selector/3 -> Product/1  "<DCM>"
  Bus Selector/2 -> Sum/1  "<Vb>"
  6DOF Bus/1 -> Bus Selector/1
  Selector/1 -> Gain_-1/1
  Gain_-1/1 -> Saturation_2/1
  Bus Selector/1 -> Selector/1  "<Xe>"
  Saturation_2/1 -> Wind Shear Model/1, Dryden Wind Turbulence Model (Discrete (-q +r))/1, Dryden Wind Turbulence Model (Discrete (-q +r))1/1
  Product1/1 -> Bus Creator/1  "Windb"
  Bus Creator/1 -> WindOut/1

== system QuadModelLib/SensorFault/GyroNoiseSwitch3 ==
  In1 : Inport
  Constant2 : Constant  Value=0.3
  Product4 : Product
  Out1 : Outport  VectorParamsAs1DForOutWhenUnconnected=off
  wires:
  Constant2/1 -> Product4/2
  Product4/1 -> Out1/1
  In1/1 -> Product4/1

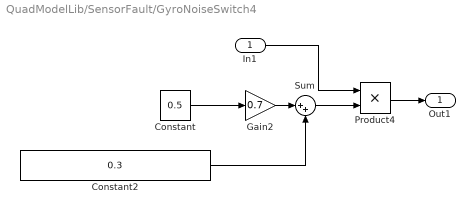
== system QuadModelLib/SensorFault/GyroNoiseSwitch4 ==
  In1 : Inport
  Constant : Constant  Value=0.5
  Constant2 : Constant  Value=0.3
  Gain2 : Gain  Gain=0.7
  Product4 : Product
  Sum : Sum  Inputs=|++
  Out1 : Outport  VectorParamsAs1DForOutWhenUnconnected=off
  wires:
  Sum/1 -> Product4/2
  Product4/1 -> Out1/1
  Gain2/1 -> Sum/1
  In1/1 -> Product4/1
  Constant2/1 -> Sum/2
  Constant/1 -> Gain2/1

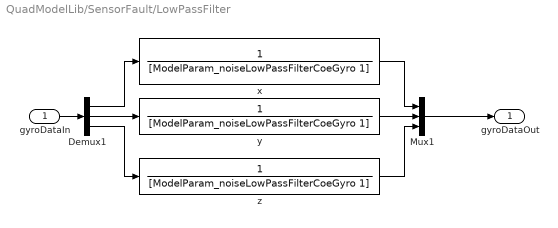
== system QuadModelLib/SensorFault/LowPassFilter ==
  gyroDataIn : Inport
  Demux1 : Demux  Outputs=3
  Mux1 : Mux  Inputs=3
  x : TransferFcn  Denominator=[ModelParam_noiseLowPassFilterCoeGyro 1]
  y : TransferFcn  Denominator=[ModelParam_noiseLowPassFilterCoeGyro 1]
  z : TransferFcn  Denominator=[ModelParam_noiseLowPassFilterCoeGyro 1]
  gyroDataOut : Outport  VectorParamsAs1DForOutWhenUnconnected=off
  wires:
  Mux1/1 -> gyroDataOut/1
  z/1 -> Mux1/3
  x/1 -> Mux1/1
  Demux1/1 -> x/1
  y/1 -> Mux1/2
  gyroDataIn/1 -> Demux1/1
  Demux1/2 -> y/1
  Demux1/3 -> z/1

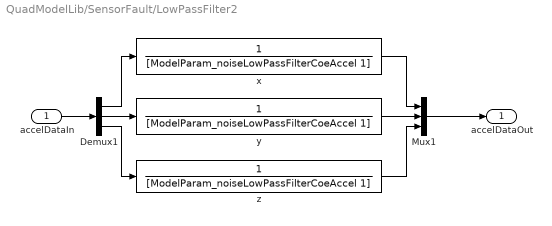
== system QuadModelLib/SensorFault/LowPassFilter2 ==
  accelDataIn : Inport
  Demux1 : Demux  Outputs=3
  Mux1 : Mux  Inputs=3
  x : TransferFcn  Denominator=[ModelParam_noiseLowPassFilterCoeAccel 1]
  y : TransferFcn  Denominator=[ModelParam_noiseLowPassFilterCoeAccel 1]
  z : TransferFcn  Denominator=[ModelParam_noiseLowPassFilterCoeAccel 1]
  accelDataOut : Outport  VectorParamsAs1DForOutWhenUnconnected=off
  wires:
  Mux1/1 -> accelDataOut/1
  z/1 -> Mux1/3
  x/1 -> Mux1/1
  Demux1/1 -> x/1
  y/1 -> Mux1/2
  accelDataIn/1 -> Demux1/1
  Demux1/2 -> y/1
  Demux1/3 -> z/1

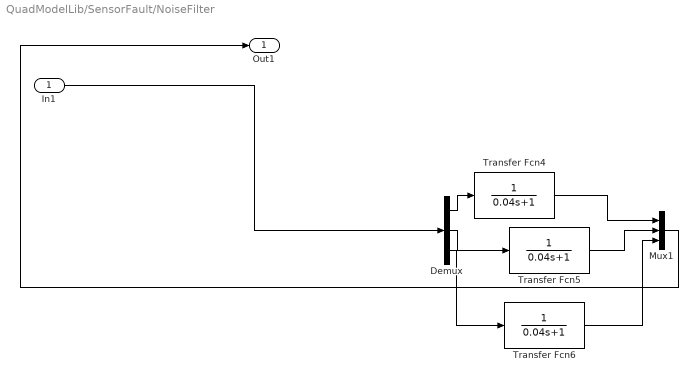
== system QuadModelLib/SensorFault/NoiseFilter ==
  In1 : Inport
  Demux : Demux  Outputs=3
  Mux1 : Mux  Inputs=3
  Transfer Fcn4 : TransferFcn  Denominator=[0.04 1]
  Transfer Fcn5 : TransferFcn  Denominator=[0.04 1]
  Transfer Fcn6 : TransferFcn  Denominator=[0.04 1]
  Out1 : Outport  VectorParamsAs1DForOutWhenUnconnected=off
  wires:
  Mux1/1 -> Out1/1
  In1/1 -> Demux/1
  Demux/3 -> Transfer Fcn6/1
  Transfer Fcn4/1 -> Mux1/1
  Transfer Fcn6/1 -> Mux1/3
  Demux/1 -> Transfer Fcn4/1
  Transfer Fcn5/1 -> Mux1/2
  Demux/2 -> Transfer Fcn5/1

== system QuadModelLib/SensorFault/NoiseFilter1 ==
  In1 : Inport
  Demux : Demux  Outputs=3
  Mux1 : Mux  Inputs=3
  Transfer Fcn4 : TransferFcn  Denominator=[0.04 1]
  Transfer Fcn5 : TransferFcn  Denominator=[0.04 1]
  Transfer Fcn6 : TransferFcn  Denominator=[0.04 1]
  Out1 : Outport  VectorParamsAs1DForOutWhenUnconnected=off
  wires:
  Mux1/1 -> Out1/1
  In1/1 -> Demux/1
  Demux/3 -> Transfer Fcn6/1
  Transfer Fcn4/1 -> Mux1/1
  Transfer Fcn6/1 -> Mux1/3
  Demux/1 -> Transfer Fcn4/1
  Transfer Fcn5/1 -> Mux1/2
  Demux/2 -> Transfer Fcn5/1

== system QuadModelLib/SensorFault/NoiseFilter2 ==
  In1 : Inport
  Demux : Demux  Outputs=3
  Mux1 : Mux  Inputs=3
  Transfer Fcn4 : TransferFcn  Denominator=[0.05 1]
  Transfer Fcn5 : TransferFcn  Denominator=[0.05 1]
  Transfer Fcn6 : TransferFcn  Denominator=[0.05 1]
  Out1 : Outport  VectorParamsAs1DForOutWhenUnconnected=off
  wires:
  Mux1/1 -> Out1/1
  In1/1 -> Demux/1
  Demux/3 -> Transfer Fcn6/1
  Transfer Fcn4/1 -> Mux1/1
  Transfer Fcn6/1 -> Mux1/3
  Demux/1 -> Transfer Fcn4/1
  Transfer Fcn5/1 -> Mux1/2
  Demux/2 -> Transfer Fcn5/1

== matlab function QuadModelLib/SensorFault/FaultParamsExtract2 ==
  settings: updateMethod=DISCRETE
  data: FaultID input; inInts input; hasFault_mag output; inFloats input; FaultParam output
function [hasFault_mag, FaultParam] = fcn(FaultID,inInts,inFloats)
persistent hFault;
persistent fParam;

if isempty(hFault)
    hFault=false;
end
if isempty(fParam)
    fParam=zeros(20,1);
end

hFaultTmp=false;
fParamTmp=zeros(20,1);
j=1;
for i=1:8
    if inInts(i) == FaultID
        hFaultTmp=true;
        fParamTmp(2*j-1)=inFloats(2*i-1);
        fParamTmp(2*j)=inFloats(2*i);
        j=j+1;
    end
end
if hFaultTmp
    hFault=hFaultTmp;
    fParamTmp(17:20) = inFloats(17:20);
    fParam=fParamTmp;
end

hasFault_mag=hFault;
FaultParam=fParam;

== matlab function QuadModelLib/SensorFault/FaultParamsExtract3 ==
  settings: updateMethod=DISCRETE
  data: FaultID input; inInts input; hasFault_baro output; inFloats input; FaultParam output
function [hasFault_baro, FaultParam] = fcn(FaultID,inInts,inFloats)
persistent hFault;
persistent fParam;

if isempty(hFault)
    hFault=false;
end
if isempty(fParam)
    fParam=zeros(20,1);
end

hFaultTmp=false;
fParamTmp=zeros(20,1);
j=1;
for i=1:8
    if inInts(i) == FaultID
        hFaultTmp=true;
        fParamTmp(2*j-1)=inFloats(2*i-1);
        fParamTmp(2*j)=inFloats(2*i);
        j=j+1;
    end
end
if hFaultTmp
    hFault=hFaultTmp;
    fParamTmp(17:20) = inFloats(17:20);
    fParam=fParamTmp;
end

hasFault_baro=hFault;
FaultParam=fParam;

== matlab function QuadModelLib/WindFault/TurbWindStrength_Dec_Switch ==
  data: vwind input size=3; TurbWind output size=3; TurbWindParams input
function TurbWind = fcn(vwind,TurbWindParams)

TurbWind=vwind*TurbWindParams(1);

== matlab function QuadModelLib/SensorFault/Acc NoiseFun ==
  settings: updateMethod=DISCRETE
  data: AccIn input; y output; isAccFault input; AccFaultParams input
function y = AccFaultFun(AccIn,isAccFault,AccFaultParams)
    y = AccIn;
    
    if isAccFault
        % FaultParams(1)为标志位
        flag = AccFaultParams(1);
        
        % 覆盖模式，当为-1时，保持原有输出
        if flag == 1
            for ind = 1:3
                if AccFaultParams(ind+1) ~= -1
                    y(ind) = AccFaultParams(ind+1);
                end
            end
        
        % 叠加模式，当为-1时，保持原有输出
        elseif flag == 2
            for ind = 1:3
                if AccFaultParams(ind+1) ~= -1
                    y(ind) = y(ind) + AccFaultParams(ind+1);
                end
            end

        % 噪声模式，当为-1时，保持原有输出
        elseif flag == 3
            mean = AccFaultParams(2);
            stddev = AccFaultParams(3);
            for ind = 1:3
                if AccFaultParams(ind+3) ~= -1
                    y(ind) = y(ind) + generate_wgn(mean,stddev);
                end
            end

        % 尺度因子模式，当为-1时，保持原有输出
        elseif flag == 4
            for ind = 1:3
                if AccFaultParams(ind+1) ~= -1
                    y(ind) = y(ind) * AccFaultParams(ind+1);
                end
            end
        end

    end

end

function y = generate_wgn(mean,stddev)
    persistent V1 V2 S phase

    if isempty(phase)
        phase = true;
        V1 = 0; 
        V2 = 0; 
        S = 0; 
    end
    
    if phase
        while true
            U1 = rand();
            U2 = rand();
            V1 = 2.0 * U1 - 1.0;
            V2 = 2.0 * U2 - 1.0;
            S = V1 * V1 + V2 * V2;
            if S < 1.0 && abs(S) >= 1e-8
                break;
            end
        end
        X = V1 * sqrt(-2.0 * log(S) / S);
    else
        X = V2 * sqrt(-2.0 * log(S) / S);
    end
    
    y = mean + stddev * X;
  
    phase = ~phase;

end

== matlab function QuadModelLib/WindFault/SheerWindStrength_Dec_Switch ==
  data: vwind input; SheerWind output; SheerWindParams input
function SheerWind = fcn(vwind,SheerWindParams)
SheerWind=vwind*SheerWindParams(1);

== matlab function QuadModelLib/BatteryFault/FaultParamsExtract ==
  settings: updateMethod=DISCRETE
  data: FaultID input; inInts input; hasFault_isUseCustomHovTime output; inFloats input; UserCustomFaultParam output
function [hasFault_isUseCustomHovTime, UserCustomFaultParam] = fcn(FaultID,inInts,inFloats)
persistent hFault;
persistent fParam;

if isempty(hFault)
    hFault=false;
end
if isempty(fParam)
    fParam=zeros(20,1);
end

hFaultTmp=false;
fParamTmp=zeros(20,1);
j=1;
for i=1:8
    if inInts(i) == FaultID
        hFaultTmp=true;
        fParamTmp(2*j-1)=inFloats(2*i-1);
        fParamTmp(2*j)=inFloats(2*i);
        j=j+1;
    end
end
if hFaultTmp
    hFault=hFaultTmp;
    fParamTmp(17:20) = inFloats(17:20);
    fParam=fParamTmp;
end

hasFault_isUseCustomHovTime=hFault;
UserCustomFaultParam=fParam;

== matlab function QuadModelLib/SensorFault/Gyro NoiseFun ==
  settings: updateMethod=DISCRETE
  data: GyroIn input; y output; isGyroFault input; GyroFaultParams input
function y = GyroFaultFun(GyroIn,isGyroFault,GyroFaultParams)
    y = GyroIn;
    
    if isGyroFault
        % FaultParams(1)为标志位
        flag = GyroFaultParams(1);
        
        % 覆盖模式，当为-1时，保持原有输出
        if flag == 1
            for ind = 1:3
                if GyroFaultParams(ind+1) ~= -1
                    y(ind) = GyroFaultParams(ind+1);
                end
            end
        
        % 叠加模式，当为-1时，保持原有输出
        elseif flag == 2
            for ind = 1:3
                if GyroFaultParams(ind+1) ~= -1
                    y(ind) = y(ind) + GyroFaultParams(ind+1);
                end
            end

        % 噪声模式，当为-1时，保持原有输出
        elseif flag == 3
            mean = GyroFaultParams(2);
            stddev = GyroFaultParams(3);
            for ind = 1:3
                if GyroFaultParams(ind+3) ~= -1
                    y(ind) = y(ind) + generate_wgn(mean,stddev);
                end
            end

        % 尺度因子模式，当为-1时，保持原有输出
        elseif flag == 4
            for ind = 1:3
                if GyroFaultParams(ind+1) ~= -1
                    y(ind) = y(ind) * GyroFaultParams(ind+1);
                end
            end
        end

    end

end

function y = generate_wgn(mean,stddev)
    persistent V1 V2 S phase

    if isempty(phase)
        phase = true;
        V1 = 0; 
        V2 = 0; 
        S = 0; 
    end
    
    if phase
        while true
            U1 = rand();
            U2 = rand();
            V1 = 2.0 * U1 - 1.0;
            V2 = 2.0 * U2 - 1.0;
            S = V1 * V1 + V2 * V2;
            if S < 1.0 && abs(S) >= 1e-8
                break;
            end
        end
        X = V1 * sqrt(-2.0 * log(S) / S);
    else
        X = V2 * sqrt(-2.0 * log(S) / S);
    end
    
    y = mean + stddev * X;
  
    phase = ~phase;

end

== matlab function QuadModelLib/SensorFault/Mag NoiseFun ==
  settings: updateMethod=DISCRETE
  data: MagIn input; isMagFault input; y output; MagFaultParams input
function y = MagFaultFun(MagIn,isMagFault,MagFaultParams)
    y = MagIn;
    
    if isMagFault
        % FaultParams(1)为标志位
        flag = MagFaultParams(1);
        
        % 覆盖模式，当为-1时，保持原有输出
        if flag == 1
            for ind = 1:3
                if MagFaultParams(ind+1) ~= -1
                    y(ind) = MagFaultParams(ind+1);
                end
            end
        
        % 叠加模式，当为-1时，保持原有输出
        elseif flag == 2
            for ind = 1:3
                if MagFaultParams(ind+1) ~= -1
                    y(ind) = y(ind) + MagFaultParams(ind+1);
                end
            end

        % 噪声模式，当为-1时，保持原有输出
        elseif flag == 3
            mean = MagFaultParams(2);
            stddev = MagFaultParams(3);
            for ind = 1:3
                if MagFaultParams(ind+3) ~= -1
                    y(ind) = y(ind) + generate_wgn(mean,stddev);
                end
            end

        % 尺度因子模式，当为-1时，保持原有输出
        elseif flag == 4
            for ind = 1:3
                if MagFaultParams(ind+1) ~= -1
                    y(ind) = y(ind) * MagFaultParams(ind+1);
                end
            end
        end

    end

end

function y = generate_wgn(mean,stddev)
    persistent V1 V2 S phase

    if isempty(phase)
        phase = true;
        V1 = 0; 
        V2 = 0; 
        S = 0; 
    end
    
    if phase
        while true
            U1 = rand();
            U2 = rand();
            V1 = 2.0 * U1 - 1.0;
            V2 = 2.0 * U2 - 1.0;
            S = V1 * V1 + V2 * V2;
            if S < 1.0 && abs(S) >= 1e-8
                break;
            end
        end
        X = V1 * sqrt(-2.0 * log(S) / S);
    else
        X = V2 * sqrt(-2.0 * log(S) / S);
    end
    
    y = mean + stddev * X;
  
    phase = ~phase;

end

== matlab function QuadModelLib/LoadFault/FaultParamsExtract1 ==
  settings: updateMethod=DISCRETE
  data: FaultID input; inInts input; hasFault_isloadShift output; inFloats input; LoadShiftFaultParam output
function [hasFault_isloadShift, LoadShiftFaultParam] = fcn(FaultID,inInts,inFloats)
persistent hFault;
persistent fParam;

if isempty(hFault)
    hFault=false;
end
if isempty(fParam)
    fParam=zeros(20,1);
end

hFaultTmp=false;
fParamTmp=zeros(20,1);
j=1;
for i=1:8
    if inInts(i) == FaultID
        hFaultTmp=true;
        fParamTmp(2*j-1)=inFloats(2*i-1);
        fParamTmp(2*j)=inFloats(2*i);
        j=j+1;
    end
end
if hFaultTmp
    hFault=hFaultTmp;
    fParamTmp(17:20) = inFloats(17:20);
    fParam=fParamTmp;
end

hasFault_isloadShift=hFault;
LoadShiftFaultParam=fParam;

== matlab function QuadModelLib/GPSFault/FaultParamsExtract ==
  settings: updateMethod=DISCRETE
  data: FaultID input; inInts input; hasFault_GPS output; inFloats input; FaultParam output
function [hasFault_GPS, FaultParam] = fcn(FaultID,inInts,inFloats)
persistent hFault;
persistent fParam;

if isempty(hFault)
    hFault=false;
end
if isempty(fParam)
    fParam=zeros(20,1);
end

hFaultTmp=false;
fParamTmp=zeros(20,1);
j=1;
for i=1:8
    if inInts(i) == FaultID
        hFaultTmp=true;
        fParamTmp(2*j-1)=inFloats(2*i-1);
        fParamTmp(2*j)=inFloats(2*i);
        j=j+1;
    end
end
if hFaultTmp
    hFault=hFaultTmp;
    fParamTmp(17:20) = inFloats(17:20);
    fParam=fParamTmp;
end

hasFault_GPS=hFault;
FaultParam=fParam;

== matlab function QuadModelLib/WindFault/noiseUpperWindBodySwitch ==
  data: NoiseParams input; y output; Noise input; isNoiseFault input
function y = fcn(NoiseParams,Noise,isNoiseFault)

y = [0;0;0];
if isNoiseFault
    Param_GlobalNoiseGainSwitch=NoiseParams(1);
    y=Noise* Param_GlobalNoiseGainSwitch;
end

== matlab function QuadModelLib/MotorFault/MotorFaultModel ==
  settings: updateMethod=DISCRETE
  data: PWMIn input; y output; isMotorFault input; MotorFaultParams input; motNum input
function y = MotorFaultFun(PWMIn,isMotorFault,MotorFaultParams,motNum)
    y = PWMIn;

    if motNum<1
        motNum=int32(1);
    end
    
    if motNum>8
        motNum=int32(8);
    end
    
    if isMotorFault
        % FaultParams(1)为标志位
        flag = MotorFaultParams(1);
        
        % 覆盖模式，当为-1时，保持原有输出
        if flag == 1
            for ind = 1:motNum
                if MotorFaultParams(ind+1) ~= -1
                    y(ind) = MotorFaultParams(ind+1);
                end
            end
        
        % 叠加模式，当为-1时，保持原有输出
        elseif flag == 2
            for ind = 1:motNum
                if MotorFaultParams(ind+1) ~= -1
                    y(ind) = y(ind) + MotorFaultParams(ind+1);
                end
            end

        % 噪声模式，当为-1时，保持原有输出
        elseif flag == 3
            mean = MotorFaultParams(2);
            stddev = MotorFaultParams(3);
            for ind = 1:motNum
                if MotorFaultParams(ind+3) ~= -1
                    y(ind) = y(ind) + generate_wgn(mean,stddev);
                end
            end

        % 尺度因子模式，当为-1时，保持原有输出
        elseif flag == 4
            for ind = 1:motNum
                if MotorFaultParams(ind+1) ~= -1
                    y(ind) = y(ind) * MotorFaultParams(ind+1);
                end
            end
        end

    end

end

function y = generate_wgn(mean,stddev)
    persistent V1 V2 S phase

    if isempty(phase)
        phase = true;
        V1 = 0; 
        V2 = 0; 
        S = 0; 
    end
    
    if phase
        while true
            U1 = rand();
            U2 = rand();
            V1 = 2.0 * U1 - 1.0;
            V2 = 2.0 * U2 - 1.0;
            S = V1 * V1 + V2 * V2;
            if S < 1.0 && abs(S) >= 1e-8
                break;
            end
        end
        X = V1 * sqrt(-2.0 * log(S) / S);
    else
        X = V2 * sqrt(-2.0 * log(S) / S);
    end
    
    y = mean + stddev * X;
  
    phase = ~phase;

end

== matlab function QuadModelLib/PropFault/FaultParamsExtract ==
  settings: updateMethod=DISCRETE
  data: FaultID input; inInts input; hasFault output; inFloats input; FaultParam output
function [hasFault, FaultParam] = fcn(FaultID,inInts,inFloats)
persistent hFault;
persistent fParam;

if isempty(hFault)
    hFault=false;
end
if isempty(fParam)
    fParam=zeros(20,1);
end

hFaultTmp=false;
fParamTmp=zeros(20,1);
j=1;
for i=1:8
    if inInts(i) == FaultID
        hFaultTmp=true;
        fParamTmp(2*j-1)=inFloats(2*i-1);
        fParamTmp(2*j)=inFloats(2*i);
        j=j+1;
    end
end
if hFaultTmp
    hFault=hFaultTmp;
    fParamTmp(17:20) = inFloats(17:20);
    fParam=fParamTmp;
end

hasFault=hFault;
FaultParam=fParam;

== matlab function QuadModelLib/PropFault/PropFaultModel ==
  settings: updateMethod=DISCRETE
  data: hasFault input; y output; FaultParam input; inPWMs input; PropNum input; unused input
function y = fcn(hasFault,FaultParam,inPWMs,PropNum,~)
% 本模块需要用到8维FaultParam的输入
%因此故障ID的格式应该是：
%inSILInts=[FaultID FaultID FaultID FaultID ...]
%inSILInts=[param1 param2 param3 param4 param5 param6 param7 param8 ...] -> FaultParam
% param的每一位表示本电机的健康系数（0到1），实际上就是pwm_out = pwm_in * param
% 如果param1=0，则电机1直接坏掉，始终输出0

y=inPWMs; %默认情况下不注入故障，直接将数据输出

if PropNum<1
    PropNum=int32(1);
end

if PropNum>8
    PropNum=int32(8);
end

if hasFault %如果注入了故障
    for i=1:PropNum
        % y(i) = inPWMs(i) * FaultParam(i)+ noise;
        y(i) = inPWMs(i) * FaultParam(i);
    end
    
end

== matlab function QuadModelLib/BatteryFault/FaultParamsExtract2 ==
  settings: updateMethod=DISCRETE
  data: FaultID input; inInts input; hasFault_isLowVoltage output; inFloats input; LowVoltageFaultParam output
function [hasFault_isLowVoltage, LowVoltageFaultParam] = fcn(FaultID,inInts,inFloats)
persistent hFault;
persistent fParam;

if isempty(hFault)
    hFault=false;
end
if isempty(fParam)
    fParam=zeros(20,1);
end

hFaultTmp=false;
fParamTmp=zeros(20,1);
j=1;
for i=1:8
    if inInts(i) == FaultID
        hFaultTmp=true;
        fParamTmp(2*j-1)=inFloats(2*i-1);
        fParamTmp(2*j)=inFloats(2*i);
        j=j+1;
    end
end
if hFaultTmp
    hFault=hFaultTmp;
    fParamTmp(17:20) = inFloats(17:20);
    fParam=fParamTmp;
end

hasFault_isLowVoltage=hFault;
LowVoltageFaultParam=fParam;

== matlab function QuadModelLib/BatteryFault/FaultParamsExtract3 ==
  settings: updateMethod=DISCRETE
  data: FaultID input; inInts input; hasFault_islowCapacity output; inFloats input; LowCapFaultParam output
function [hasFault_islowCapacity, LowCapFaultParam] = fcn(FaultID,inInts,inFloats)
persistent hFault;
persistent fParam;

if isempty(hFault)
    hFault=false;
end
if isempty(fParam)
    fParam=zeros(20,1);
end

hFaultTmp=false;
fParamTmp=zeros(20,1);
j=1;
for i=1:8
    if inInts(i) == FaultID
        hFaultTmp=true;
        fParamTmp(2*j-1)=inFloats(2*i-1);
        fParamTmp(2*j)=inFloats(2*i);
        j=j+1;
    end
end
if hFaultTmp
    hFault=hFaultTmp;
    fParamTmp(17:20) = inFloats(17:20);
    fParam=fParamTmp;
end

hasFault_islowCapacity=hFault;
LowCapFaultParam=fParam;

== matlab function QuadModelLib/SensorFault/FaultParamsExtract ==
  settings: updateMethod=DISCRETE
  data: FaultID input; inInts input; hasFault_acc output; inFloats input; FaultParam output
function [hasFault_acc, FaultParam] = fcn(FaultID,inInts,inFloats)
persistent hFault;
persistent fParam;

if isempty(hFault)
    hFault=false;
end
if isempty(fParam)
    fParam=zeros(20,1);
end

hFaultTmp=false;
fParamTmp=zeros(20,1);
j=1;
for i=1:8
    if inInts(i) == FaultID
        hFaultTmp=true;
        fParamTmp(2*j-1)=inFloats(2*i-1);
        fParamTmp(2*j)=inFloats(2*i);
        j=j+1;
    end
end
if hFaultTmp
    hFault=hFaultTmp;
    fParamTmp(17:20) = inFloats(17:20);
    fParam=fParamTmp;
end

hasFault_acc=hFault;
FaultParam=fParam;

== matlab function QuadModelLib/LoadFault/FaultParamsExtract3 ==
  settings: updateMethod=DISCRETE
  data: FaultID input; inInts input; hasFault_isloadFall output; inFloats input; LoadFallFaultParam output
function [hasFault_isloadFall, LoadFallFaultParam] = fcn(FaultID,inInts,inFloats)
persistent hFault;
persistent fParam;

if isempty(hFault)
    hFault=false;
end
if isempty(fParam)
    fParam=zeros(20,1);
end

hFaultTmp=false;
fParamTmp=zeros(20,1);
j=1;
for i=1:8
    if inInts(i) == FaultID
        hFaultTmp=true;
        fParamTmp(2*j-1)=inFloats(2*i-1);
        fParamTmp(2*j)=inFloats(2*i);
        j=j+1;
    end
end
if hFaultTmp
    hFault=hFaultTmp;
    fParamTmp(17:20) = inFloats(17:20);
    fParam=fParamTmp;
end

hasFault_isloadFall=hFault;
LoadFallFaultParam=fParam;

== matlab function QuadModelLib/LoadFault/FaultParamsExtract2 ==
  settings: updateMethod=DISCRETE
  data: FaultID input; inInts input; hasFault_isloadLeak output; inFloats input; LoadleakFaultParam output
function [hasFault_isloadLeak, LoadleakFaultParam] = fcn(FaultID,inInts,inFloats)
persistent hFault;
persistent fParam;

if isempty(hFault)
    hFault=false;
end
if isempty(fParam)
    fParam=zeros(20,1);
end

hFaultTmp=false;
fParamTmp=zeros(20,1);
j=1;
for i=1:8
    if inInts(i) == FaultID
        hFaultTmp=true;
        fParamTmp(2*j-1)=inFloats(2*i-1);
        fParamTmp(2*j)=inFloats(2*i);
        j=j+1;
    end
end
if hFaultTmp
    hFault=hFaultTmp;
    fParamTmp(17:20) = inFloats(17:20);
    fParam=fParamTmp;
end

hasFault_isloadLeak=hFault;
LoadleakFaultParam=fParam;

== matlab function QuadModelLib/WindFault/FaultParamsExtract ==
  settings: updateMethod=DISCRETE
  data: FaultID input; inInts input; hasFault_ConstWind output; inFloats input; FaultParam output
function [hasFault_ConstWind, FaultParam] = fcn(FaultID,inInts,inFloats)
persistent hFault;
persistent fParam;

if isempty(hFault)
    hFault=false;
end
if isempty(fParam)
    fParam=zeros(20,1);
end

hFaultTmp=false;
fParamTmp=zeros(20,1);
j=1;
for i=1:8
    if inInts(i) == FaultID
        hFaultTmp=true;
        fParamTmp(2*j-1)=inFloats(2*i-1);
        fParamTmp(2*j)=inFloats(2*i);
        j=j+1;
    end
end
if hFaultTmp
    hFault=hFaultTmp;
    fParamTmp(17:20) = inFloats(17:20);
    fParam=fParamTmp;
end

hasFault_ConstWind=hFault;
FaultParam=fParam;

== matlab function QuadModelLib/WindFault/FaultParamsExtract2 ==
  settings: updateMethod=DISCRETE
  data: FaultID input; inInts input; hasFault_TurbWind output; inFloats input; FaultParam output
function [hasFault_TurbWind, FaultParam] = fcn(FaultID,inInts,inFloats)
persistent hFault;
persistent fParam;

if isempty(hFault)
    hFault=false;
end
if isempty(fParam)
    fParam=zeros(20,1);
end

hFaultTmp=false;
fParamTmp=zeros(20,1);
j=1;
for i=1:8
    if inInts(i) == FaultID
        hFaultTmp=true;
        fParamTmp(2*j-1)=inFloats(2*i-1);
        fParamTmp(2*j)=inFloats(2*i);
        j=j+1;
    end
end
if hFaultTmp
    hFault=hFaultTmp;
    fParamTmp(17:20) = inFloats(17:20);
    fParam=fParamTmp;
end

hasFault_TurbWind=hFault;
FaultParam=fParam;

== matlab function QuadModelLib/WindFault/FaultParamsExtract3 ==
  settings: updateMethod=DISCRETE
  data: FaultID input; inInts input; hasFault_SheerWind output; inFloats input; FaultParam output
function [hasFault_SheerWind, FaultParam] = fcn(FaultID,inInts,inFloats)
persistent hFault;
persistent fParam;

if isempty(hFault)
    hFault=false;
end
if isempty(fParam)
    fParam=zeros(20,1);
end

hFaultTmp=false;
fParamTmp=zeros(20,1);
j=1;
for i=1:8
    if inInts(i) == FaultID
        hFaultTmp=true;
        fParamTmp(2*j-1)=inFloats(2*i-1);
        fParamTmp(2*j)=inFloats(2*i);
        j=j+1;
    end
end
if hFaultTmp
    hFault=hFaultTmp;
    fParamTmp(17:20) = inFloats(17:20);
    fParam=fParamTmp;
end

hasFault_SheerWind=hFault;
FaultParam=fParam;
